simulink model "entry_during_exit_Actions"  (R2018b)
settings: Solver=FixedStepDiscrete  StartTime=0.0  StopTime=12  FixedStep=0.5  RelTol=1e-3
libraries: simulink x1
settings Model: Creator=marwan  LastModifiedBy=marwan

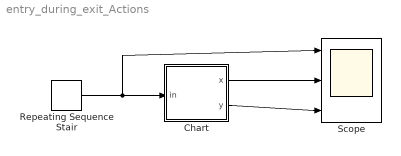
== system entry_during_exit_Actions ==
  Chart : Stateflow chart  TreatAsAtomicUnit=on
  Repeating Sequence Stair : simulink/Sources/Repeating Sequence Stair  OutValues=[2 4 6 8 10 12 14]  tsamp=-1  OutMin=[]  OutMax=[]  OutDataTypeStr=double  OutputDataTypeScalingMode=double  OutDataType=fixdt(0,8)  ConRadixGroup=Best Precision: Vector-wise  OutScaling=2^-12
  Scope : Scope  NumInputPorts=3
  wires:
  Repeating Sequence Stair/1 -> Scope/1, Chart/1(in)
  Chart/1(x) -> Scope/2
  Chart/2(y) -> Scope/3

== stateflow chart entry_during_exit_Actions/Chart ==
  state st_1
    en: x=1;
    du: x=2;
    ex: x=3;
  state st_2
    en: y=4;
    du: y=5;
    ex: y=6;
  (default) -> st_1
  st_1 -> (junction 5) : [in>5]
  (junction 5) -> st_2 : [in>10]
  st_2 -> st_1 : [in<5]
  data: in input; x output; y output
